simulink model "OCTModel_for_lin"  (R2020a)
settings: Solver=ode23t  StartTime=0.0  StopTime=simParams.duration.Value  FixedStep=0.1  MaxStep=0.1*sqrt(simParams.lengthScaleFactor.Value)  RelTol=1e-3  AbsTol=1e-3
undefined symbols (not defined in the file): ctrlFreeze, ctrlFreezeTime, exit, flowDir, linCtrl, rampSlope, trimCtrl
libraries: simulink x3, sharedutil x3, environment_cl x1, flightController_cl x1, gndStnController_cl x1, hiLvlController_cl x1, plant_cl x1, sensorProcessing_cl x1, sensors_cl x1
PreSaveFcn:
  | % Callback to reset the view so that the
  | % the next person to open isn't totally lost.
  | hilite_system('OCTModel_for_lin/plant');
  | hilite_system('OCTModel_for_lin/plant','none');
  | set_param(gcs,'Zoomfactor','fit to view')
settings Model: SimulationMode=accelerator  ExtModeTrigDuration=100  Creator=mcobb  LastModifiedBy=andre
settings SolverCC: AlgebraicLoopSolver=LineSearch  SolverResetMethod=Robust
settings DataIOCC: ExternalInput=[0 0 0 0 0 0]  InitialState=[]  LoadExternalInput=on  LoadInitialState=on  SaveFinalState=on  SaveFormat=Structure  SaveOutput=off  SaveState=on  DSMLogging=off  ReturnWorkspaceOutputs=off  StateSaveName=tmp_raccel_xout
settings OptimizationCC: DefaultParameterBehavior=Inlined  BufferReuse=off  EfficientMapNaN2IntZero=off
settings DebuggingCC: SignalRangeChecking=error  AlgebraicLoopMsg=none  ArtificialAlgebraicLoopMsg=none  InitInArrayFormatMsg=none  ArithmeticOperatorsInVariantConditions=warning
settings HardwareCC: TargetBitPerPointer=64  TargetBitPerSizeT=64  TargetBitPerPtrDiffT=64  TargetLongLongMode=on  TargetIntDivRoundTo=Zero  TargetEndianess=LittleEndian  TargetWordSize=64  TargetHWDeviceType=MATLAB Host  ProdEqTarget=off
settings SFSimCC: CustomCodeUndefinedFunction=UseInterfaceOnly
settings CodeAppCC: MaxIdLength=128
settings GRTTargetCC: TargetLangStandard=C89/C90 (ANSI)  CombineOutputUpdateFcns=off  GRTInterface=on

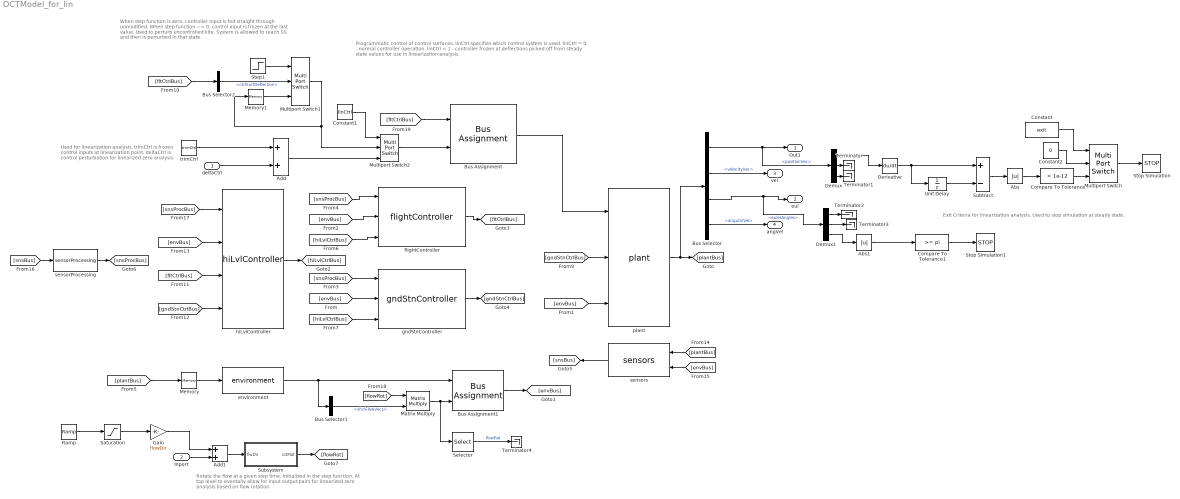
== system OCTModel_for_lin ==
  note: When step function is zero, controller input is fed straight through
      | unmodified. When step function ~= 0, control input is frozen at the
      | last value. Used to perturb uncontrolled kite. System is allowed to
      | reach SS and then is perturbed in that state.
  note: Used for linearization analysis. trimCtrl is
      | frozen control inputs at linearization point.
      | deltaCtrl is control perturbation for linearized
      | zero analysis.
  note: Programmatic control of control surfaces. linCtrl specifies which control  system is used.
      | linCtrl = 0 - normal controller operation. linCtrl = 1 - controller frozen at deflections picked off
      | from steady state values for use in linearization analysis.
  note: Exit Criteria for linearization analysis. Used to stop simulation at steady state.
  note: Rotate the flow at a given step time. Initialized in the step function.
      | At top level to eventally allow for input output pairs
      |  for linearized zero analysis based on flow rotation
  deltaCtrl : Inport  PortDimensions=4
  Inport : Inport  Port=2  PortDimensions=1
  Abs : Abs  ZeroCross=off
  Abs1 : Abs
  Add : Sum
  Add1 : Sum
  Bus Assignment : BusAssignment  AssignedSignals=ctrlSurfDeflection
  Bus Assignment1 : BusAssignment  AssignedSignals=vhclFlowVecs
  Bus Selector : BusSelector  OutputSignals=positionVec,velocityVec,eulerAngles,angularVel
  Bus Selector1 : BusSelector  OutputSignals=vhclFlowVecs
  Bus Selector2 : BusSelector  OutputSignals=ctrlSurfDeflection
  Compare To Tolerance : simulink/Logic and Bit Operations/Compare To Constant  relop=<  const=1e-12  OutDataTypeStr=boolean  ZeroCross=off
  Compare To Tolerance1 : simulink/Logic and Bit Operations/Compare To Constant  relop=>=  const=pi  OutDataTypeStr=boolean  ZeroCross=off
  Constant : Constant  Value=exit
  Constant1 : Constant  Value=linCtrl
  Constant2 : Constant  Value=0
  Demux : Demux  Outputs=3
  Demux1 : Demux  Outputs=3
  Derivative : Derivative
  Gain : Gain  Gain=flowDir
  Matrix Multiply : Product  Multiplication=Matrix(*)
  Memory : Memory
  Memory1 : Memory  LinearizeMemory=on
  Multiport Switch : MultiPortSwitch  DataPortOrder=Zero-based contiguous  Inputs=2  zeroidx=on
  Multiport Switch1 : MultiPortSwitch  DataPortOrder=Zero-based contiguous  Inputs=2  zeroidx=on
  Multiport Switch2 : MultiPortSwitch  DataPortOrder=Zero-based contiguous  Inputs=2  zeroidx=on
  Ramp : simulink/Sources/Ramp  slope=rampSlope  start=stepTime  InitialOutput=0
  Saturation : Saturate  UpperLimit=1  LowerLimit=0
  Selector : Selector  NumberOfDimensions=2  InputPortWidth=3  IndexOptions=Select all,Index vector (dialog)  Indices=[1 3],5  OutputSizes=1,1
  Step1 : Step  Time=ctrlFreezeTime  After=ctrlFreeze  SampleTime=0
  Stop Simulation : Stop
  Stop Simulation1 : Stop
  Subsystem : Subsystem
  Subtract : Sum  Inputs=+-
  Terminator{,1..4} (5 alike) : Terminator
  Unit Delay : UnitDelay  InitialCondition=0.1  SampleTime=-1
  environment : environment_cl/environment  SystemSampleTime=-1  Latency=0  AutoFrameSizeCalculation=off
  flightController : flightController_cl/flightController  SystemSampleTime=-1  Latency=0  AutoFrameSizeCalculation=off
      link override slController/Gain2: Gain=-1
      link override slController/Roll Control/filteredPIDControllerRes: kp=0  ki=0  kd=0  Value=0  UpperLimit=upperLimit  LowerLimit=0
      link override slController/Yaw Control/filteredPIDControllerRes: kp=fltCtrl.rudderCmd.kp.Value  ki=fltCtrl.rudderCmd.ki.Value  kd=fltCtrl.rudderCmd.kd.Value  Value=fltCtrl.rudderCmd.tau.Value  UpperLimit=fltCtrl.controlSigMax.upperLimit.Value  LowerLimit=fltCtrl.controlSigMax.lowerLimit.Value
      link override slController/Yaw Setpoint PID Control/Gain1: Gain=-1
      link override slController/Yaw Setpoint PID Control/Saturation: UpperLimit=90  LowerLimit=-90
  gndStnController : gndStnController_cl/gndStnController  SystemSampleTime=-1  Latency=0  AutoFrameSizeCalculation=off
  hiLvlController : hiLvlController_cl/hiLvlController  SystemSampleTime=-1  Latency=0  AutoFrameSizeCalculation=off
  plant : plant_cl/plant  SystemSampleTime=-1  Latency=0  AutoFrameSizeCalculation=off
  sensorProcessing : sensorProcessing_cl/sensorProcessing  SystemSampleTime=-1  Latency=0  AutoFrameSizeCalculation=off
  sensors : sensors_cl/sensors  SystemSampleTime=-1  Latency=0  AutoFrameSizeCalculation=off
  trimCtrl : Constant  Value=trimCtrl
  Out1 : Outport
  eul : Outport  Port=2
  vel : Outport  Port=3
  angVel : Outport  Port=4
  wires:
  Memory/1 -> environment/1
  [envBus] -> gndStnController/2
  [snsProcBus] -> gndStnController/1
  [snsProcBus] -> flightController/1
  [snsProcBus] -> hiLvlController/1
  flightController/1 -> [fltCtrlBus]
  gndStnController/1 -> [gndStnCtrlBus]
  [envBus] -> hiLvlController/2
  [fltCtrlBus] -> hiLvlController/3
  [gndStnCtrlBus] -> hiLvlController/4
  [plantBus] -> Memory/1
  [hiLvlCtrlBus] -> flightController/3
  [hiLvlCtrlBus] -> gndStnController/3
  hiLvlController/1 -> [hiLvlCtrlBus]
  [envBus] -> flightController/2
  [plantBus] -> sensors/1
  [envBus] -> sensors/2
  sensors/1 -> [snsBus]
  [snsBus] -> sensorProcessing/1
  sensorProcessing/1 -> [snsProcBus]
  plant/1 -> Bus Selector/1, [plantBus]
  [gndStnCtrlBus] -> plant/2
  [envBus] -> plant/3
  Bus Selector/2 -> vel/1  "<velocityVec>"
  Bus Selector/3 -> Demux1/1, eul/1  "<eulerAngles>"
  Bus Selector/4 -> angVel/1  "<angularVel>"
  trimCtrl/1 -> Add/1
  Add/1 -> Multiport Switch2/3
  [fltCtrlBus] -> Bus Selector2/1
  environment/1 -> Bus Selector1/1, Bus Assignment1/1
  Bus Selector/1 -> Demux/1, Out1/1  "<positionVec>"
  deltaCtrl/1 -> Add/2
  Bus Selector1/1 -> Matrix Multiply/2  "<vhclFlowVecs>"
  Subsystem/1(rotMat) -> [flowRot]
  Inport/1 -> Add1/2
  [flowRot] -> Matrix Multiply/1
  Bus Assignment1/1 -> [envBus]
  Matrix Multiply/1 -> Selector/1, Bus Assignment1/2
  Add1/1 -> Subsystem/1(flwDir)
  Bus Selector2/1 -> Multiport Switch1/2  "<ctrlSurfDeflection>"
  Multiport Switch1/1 -> Memory1/1, Multiport Switch2/2
  Memory1/1 -> Multiport Switch1/3
  Step1/1 -> Multiport Switch1/1
  Constant1/1 -> Multiport Switch2/1
  [fltCtrlBus] -> Bus Assignment/1
  Multiport Switch2/1 -> Bus Assignment/2
  Demux/1 -> Derivative/1
  Compare To Tolerance/1 -> Multiport Switch/3
  Abs/1 -> Compare To Tolerance/1
  Unit Delay/1 -> Subtract/2
  Subtract/1 -> Abs/1
  Derivative/1 -> Unit Delay/1, Subtract/1
  Demux/2 -> Terminator/1
  Demux/3 -> Terminator1/1
  Bus Assignment/1 -> plant/1
  Constant/1 -> Multiport Switch/1
  Multiport Switch/1 -> Stop Simulation/1
  Constant2/1 -> Multiport Switch/2
  Gain/1 -> Add1/1
  Demux1/3 -> Abs1/1
  Abs1/1 -> Compare To Tolerance1/1
  Demux1/1 -> Terminator2/1
  Demux1/2 -> Terminator3/1
  Compare To Tolerance1/1 -> Stop Simulation1/1
  Selector/1 -> Terminator4/1  "flowRot"
  Ramp/1 -> Saturation/1
  Saturation/1 -> Gain/1

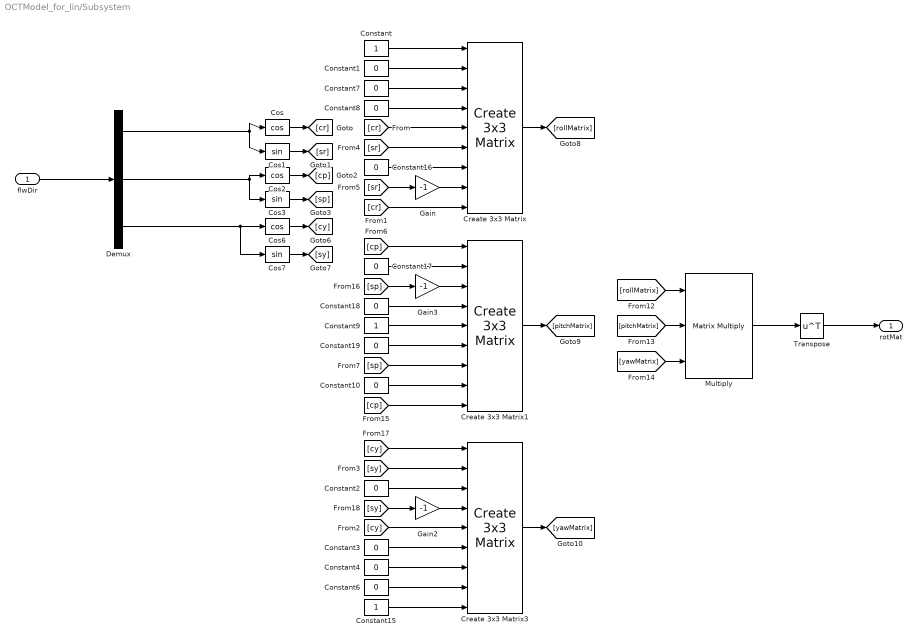
== system OCTModel_for_lin/Subsystem ==
  flwDir : Inport
  Constant : Constant
  Constant{1..4,6..8,10,16..19} (12 alike) : Constant  Value=0
  Constant15 : Constant
  Constant9 : Constant
  Cos : Trigonometry  Operator=cos
  Cos1 : Trigonometry
  Cos2 : Trigonometry  Operator=cos
  Cos3 : Trigonometry
  Cos6 : Trigonometry  Operator=cos
  Cos7 : Trigonometry
  Create 3x3 Matrix : sharedutil/Create 3x3 Matrix  aMode=aMode
  Create 3x3 Matrix1 : sharedutil/Create 3x3 Matrix  aMode=aMode
  Create 3x3 Matrix3 : sharedutil/Create 3x3 Matrix  aMode=aMode
  Demux : Demux  Outputs=3
  Gain : Gain  Gain=-1
  Gain2 : Gain  Gain=-1
  Gain3 : Gain  Gain=-1
  Multiply : Product  Inputs=3  Multiplication=Matrix(*)
  Transpose : Math  Operator=transpose  SaturateOnIntegerOverflow=on
  rotMat : Outport
  wires:
  Multiply/1 -> Transpose/1
  [pitchMatrix] -> Multiply/2
  Create 3x3 Matrix3/1 -> [yawMatrix]
  [sr] -> Gain/1
  Constant9/1 -> Create 3x3 Matrix1/5
  Gain/1 -> Create 3x3 Matrix/8
  Constant1/1 -> Create 3x3 Matrix/2
  Constant/1 -> Create 3x3 Matrix/1
  [sp] -> Gain3/1
  Constant10/1 -> Create 3x3 Matrix1/8
  [cp] -> Create 3x3 Matrix1/1
  [sy] -> Create 3x3 Matrix3/2
  Constant4/1 -> Create 3x3 Matrix3/7
  Create 3x3 Matrix1/1 -> [pitchMatrix]
  [cy] -> Create 3x3 Matrix3/1
  [rollMatrix] -> Multiply/1
  Constant17/1 -> Create 3x3 Matrix1/2
  Gain2/1 -> Create 3x3 Matrix3/4
  [sy] -> Gain2/1
  Gain3/1 -> Create 3x3 Matrix1/3
  [cr] -> Create 3x3 Matrix/9
  Constant2/1 -> Create 3x3 Matrix3/3
  Demux/1 -> Cos1/1, Cos/1
  Cos1/1 -> [sr]
  [cy] -> Create 3x3 Matrix3/5
  [yawMatrix] -> Multiply/3
  Constant6/1 -> Create 3x3 Matrix3/8
  Cos/1 -> [cr]
  [sr] -> Create 3x3 Matrix/6
  Create 3x3 Matrix/1 -> [rollMatrix]
  Constant18/1 -> Create 3x3 Matrix1/4
  Constant19/1 -> Create 3x3 Matrix1/6
  Cos6/1 -> [cy]
  [sp] -> Create 3x3 Matrix1/7
  Demux/2 -> Cos3/1, Cos2/1
  Constant8/1 -> Create 3x3 Matrix/4
  [cp] -> Create 3x3 Matrix1/9
  Demux/3 -> Cos7/1, Cos6/1
  Cos2/1 -> [cp]
  Constant3/1 -> Create 3x3 Matrix3/6
  Cos3/1 -> [sp]
  Cos7/1 -> [sy]
  Constant7/1 -> Create 3x3 Matrix/3
  Constant16/1 -> Create 3x3 Matrix/7
  [cr] -> Create 3x3 Matrix/5
  Constant15/1 -> Create 3x3 Matrix3/9
  flwDir/1 -> Demux/1
  Transpose/1 -> rotMat/1
